simulink model "UpperLimb_Planar"  (R2024b)
settings: Solver=ode45  StartTime=0.0  StopTime=T_sim  FixedStep=1e-3  MaxStep=1e-2  RelTol=1e-3
values from neighbouring files (symbols this model uses):
  activ_dyn = 1    [UpperLimbExo_Parameters.m]
  alpha0 = 180/pi*[M_CORB.alpha0; M_TMAJ.alpha0; M_DELT.alpha0; M_TRIPB.CMED.alpha0; M_TRIPB.CLAT.alpha0;  M_TRIPB.CLONG.alpha0; M_BICB.alpha0; M_BRACH.alpha0]*pi/180    [UpperLimbExo_Parameters.m]
  b12 = dampingOn*0.2    (= 0.2)    [UpperLimbExo_Parameters.m]
  b23 = dampingOn*0.2    (= 0.2)    [UpperLimbExo_Parameters.m]
  FM0 = (1-zraneni).*FM0    [UpperLimbExo_Parameters.m]
  g = 9.81    [UpperLimbExo_Parameters.m]
  I2S2 = 0.0208    [UpperLimbExo_Parameters.m]
  I3S3 = 0.006    [UpperLimbExo_Parameters.m]
  Kd = 2*sqrt(Kp)    [UpperLimbExo_Parameters.m]
  Kp = diag([400, 800])    [UpperLimbExo_Parameters.m]
  Ku = 10    [UpperLimbExo_Parameters.m]
  L2 = 0.29    [UpperLimbExo_Parameters.m]
  LM0 = RATIO.*[M_CORB.LM0; M_TMAJ.LM0; M_DELT.LM0; M_TRIPB.CMED.LM0; M_TRIPB.CLAT.LM0; M_TRIPB.CLONG.LM0; M_BICB.LM0; M_BRACH.LM0]    [UpperLimbExo_Parameters.m]
  LS2 = L2/2    (= 0.145)    [UpperLimbExo_Parameters.m]
  LS3 = LS2    (= 0.145)    [UpperLimbExo_Parameters.m]
  LTs = RATIO.*[M_CORB.LTs; M_TMAJ.LTs; M_DELT.LTs; M_TRIPB.CMED.LTs; M_TRIPB.CLAT.LTs;  M_TRIPB.CLONG.LTs; M_BICB.LTs; M_BRACH.LTs]    [UpperLimbExo_Parameters.m]
  m2 = 2.0519    [UpperLimbExo_Parameters.m]
  m3 = 0.5464 + 0.5464    (= 1.0928)    [UpperLimbExo_Parameters.m]
  T_sampleData = 1e-0    (= 1)    [UpperLimb_Main.m]
  tauA = 15/1000    (= 0.015)    [UpperLimbExo_Parameters.m]
  tauD = 50/1000    (= 0.05)    [UpperLimbExo_Parameters.m]
libraries: simulink_extras x1
settings Model: Creator=jakub  LastModifiedBy=jakub
settings DebuggingCC: ReadBeforeWriteMsg=DisableAll  WriteAfterWriteMsg=DisableAll  WriteAfterReadMsg=DisableAll  MultiTaskDSMMsg=none
settings ModelReferenceCC: UpdateModelReferenceTargets=IfOutOfDate
settings SFSimCC: SFSimEcho=off

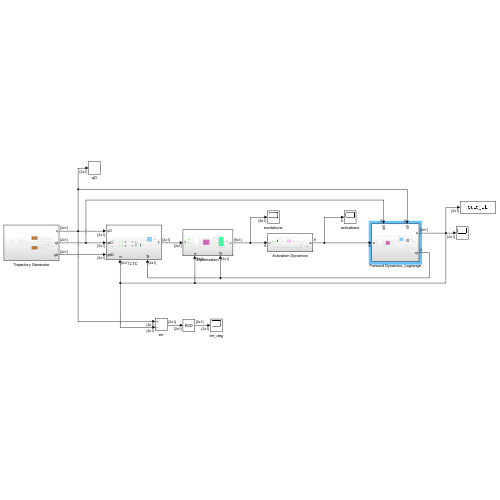
[thumbnail: Simulink's stored preview of the top-level diagram]
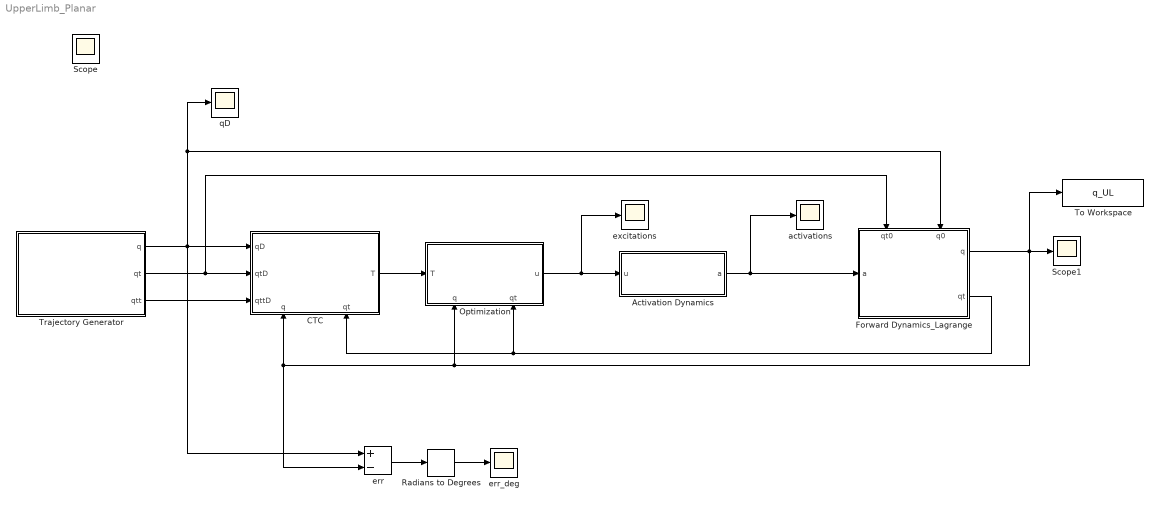
== system UpperLimb_Planar ==
  Activation Dynamics : Subsystem
  CTC : Subsystem
      settings: PortSchema="{\"entries\":[{\"content\":{\"sides\":[{\"content\":{\"connectorIds\":[\"In1\",\"In2\",\"In3\"]},\"type\":\"ConnectorPlacement.EquallySpacedRectSide\",\"uuid\":\"9771eba7-c940-48d8-8da9-6d911b5851fc\"},{\"content\":{\"connectorIds\":[\"Out1\"],\"side\":\"RIGHT\"},\"type\":\"ConnectorPlacement.EquallySpacedRectSide\",\"uuid\":\"6a59c5b5-9e25-411a-90e6-5bf21983ac5c\"},{\"content\":{\"side\":\"TOP\"},\"type\":\"ConnectorPlacement.EquallySpacedRectSide\",\"uuid\":\"c119b971-ed02-4623-8220-b75198a2fdb0\"},{\"content\":{\"connectorIds\":[\"In4\",\"In5\"],\"side\":\"BOTTOM\"},\"type\":\"ConnectorPlacement.EquallySpacedRectSide\",\"uuid\":\"c8357dcf-0796-45f4-b88a-26b4637402a4\"}]},\"type\":\"ConnectorPlacement.EquallySpacedConnector\",\"uuid\":\"a7be367e-b174-4db7-82d5-13ec9cf2ed48\"}],\"packageUris\":[\"http://schema.mathworks.com/mf0/Connector/R2020b\"],\"version\":\"1.0\"}"
  Forward Dynamics_Lagrange : Subsystem
      settings: PortSchema="{\"entries\":[{\"content\":{\"sides\":[{\"content\":{\"connectorIds\":[\"In1\"]},\"type\":\"ConnectorPlacement.EquallySpacedRectSide\",\"uuid\":\"4e4f4804-ca43-420b-a896-94143398389c\"},{\"content\":{\"connectorIds\":[\"Out1\",\"Out2\"],\"side\":\"RIGHT\"},\"type\":\"ConnectorPlacement.EquallySpacedRectSide\",\"uuid\":\"5fd0c042-4ed2-4608-8a89-d3cfef128ff0\"},{\"content\":{\"connectorIds\":[\"In2\",\"In3\"],\"side\":\"TOP\"},\"type\":\"ConnectorPlacement.EquallySpacedRectSide\",\"uuid\":\"9152b886-03a6-40db-8757-3e13ff02ab8e\"},{\"content\":{\"side\":\"BOTTOM\"},\"type\":\"ConnectorPlacement.EquallySpacedRectSide\",\"uuid\":\"2e772fd2-4f40-44b3-932b-1325c76caf16\"}]},\"type\":\"ConnectorPlacement.EquallySpacedConnector\",\"uuid\":\"c9c97ee9-fbd0-4586-b58c-f13fd24f0fc7\"}],\"packageUris\":[\"http://schema.mathworks.com/mf0/Connector/R2020b\"],\"version\":\"1.0\"}"
  Optimization : Subsystem
      settings: PortSchema="{\"entries\":[{\"content\":{\"sides\":[{\"content\":{\"connectorIds\":[\"In1\"]},\"type\":\"ConnectorPlacement.EquallySpacedRectSide\",\"uuid\":\"b44a492b-355a-41d1-979d-356380411af8\"},{\"content\":{\"connectorIds\":[\"Out1\"],\"side\":\"RIGHT\"},\"type\":\"ConnectorPlacement.EquallySpacedRectSide\",\"uuid\":\"d99b47b0-e23d-4c30-9cd9-10c88a2db076\"},{\"content\":{\"side\":\"TOP\"},\"type\":\"ConnectorPlacement.EquallySpacedRectSide\",\"uuid\":\"52778e40-0bc9-47fa-bb22-aef647873746\"},{\"content\":{\"connectorIds\":[\"In2\",\"In3\"],\"side\":\"BOTTOM\"},\"type\":\"ConnectorPlacement.EquallySpacedRectSide\",\"uuid\":\"29328456-4ee0-4f69-ade8-350b50f8103c\"}]},\"type\":\"ConnectorPlacement.EquallySpacedConnector\",\"uuid\":\"e5ef0993-fdc7-4811-bff5-ccf29bcab6f8\"}],\"packageUris\":[\"http://schema.mathworks.com/mf0/Connector/R2020b\"],\"version\":\"1.0\"}"
  Radians to Degrees : simulink_extras/Transformations/Radians to Degrees
  Scope1 : Scope
  To Workspace : ToWorkspace  VariableName=q_UL  SaveFormat=Timeseries  SampleTime=T_sampleData
  Trajectory Generator : Subsystem
  activations : Scope
  err : Sum  Inputs=+-
  err_deg : Scope
  excitations : Scope
  qD : Scope
  Scope : Scope
  wires:
  Optimization/1(u) -> Activation Dynamics/1(u), excitations/1
  CTC/1(T) -> Optimization/1(T)
  Trajectory Generator/1(q) -> CTC/1(qD), err/1, qD/1, Forward Dynamics_Lagrange/3(q0)
  Trajectory Generator/2(qt) -> CTC/2(qtD), Forward Dynamics_Lagrange/2(qt0)
  Trajectory Generator/3(qtt) -> CTC/3(qttD)
  err/1 -> Radians to Degrees/1
  Radians to Degrees/1 -> err_deg/1
  Forward Dynamics_Lagrange/1(q) -> Optimization/2(q), CTC/4(q), err/2, To Workspace/1, Scope1/1
  Forward Dynamics_Lagrange/2(qt) -> Optimization/3(qt), CTC/5(qt)
  Activation Dynamics/1(a) -> activations/1, Forward Dynamics_Lagrange/1(a)

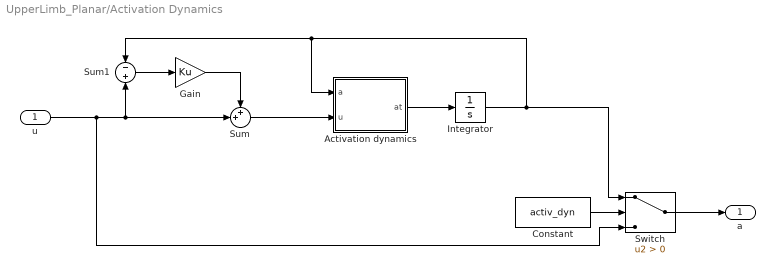
== system UpperLimb_Planar/Activation Dynamics ==
  u : Inport  OutMin=0  OutMax=1  OutDataTypeStr=double  PortDimensions=8  SampleTime=0
  Activation dynamics : MATLAB Function  TreatAsAtomicUnit=on
  Constant : Constant  Value=activ_dyn
  Gain : Gain  Gain=Ku
  Integrator : Integrator  UpperSaturationLimit=1  LowerSaturationLimit=0
  Sum : Sum  Inputs=++|
  Sum1 : Sum  Inputs=-|+
  Switch : Switch  Criteria=u2 > Threshold  ZeroCross=off  SaturateOnIntegerOverflow=off  InputSameDT=off
  a : Outport  OutMin=0  OutMax=1  OutDataTypeStr=double  PortDimensions=8  SampleTime=0
  wires:
  Sum/1 -> Activation dynamics/2(u)
  Integrator/1 -> Switch/1, Sum1/1, Activation dynamics/1(a)
  u/1 -> Sum/2, Sum1/2, Switch/3
  Constant/1 -> Switch/2
  Activation dynamics/1(at) -> Integrator/1
  Switch/1 -> a/1
  Sum1/1 -> Gain/1
  Gain/1 -> Sum/1

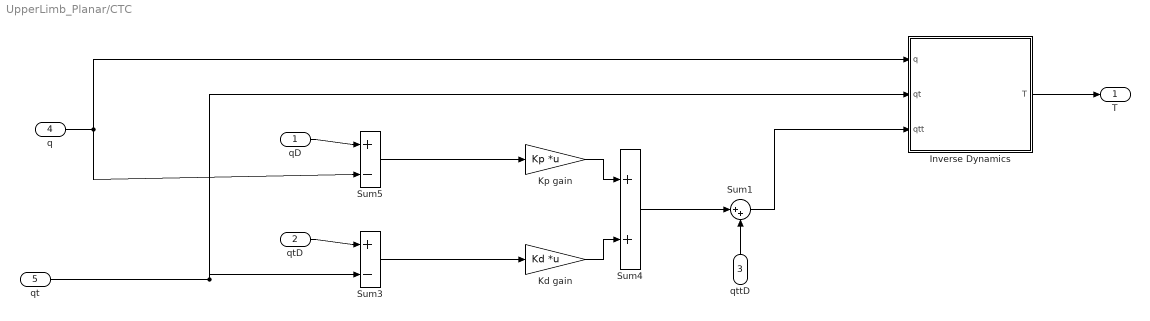
== system UpperLimb_Planar/CTC ==
  qD : Inport  OutDataTypeStr=double  Unit=rad  PortDimensions=[2 1]  SampleTime=0
  qtD : Inport  Port=2  OutDataTypeStr=double  Unit=rad/s  PortDimensions=[2 1]  SampleTime=0
  qttD : Inport  Port=3  OutDataTypeStr=double  Unit=rad/s^2  PortDimensions=[2 1]  SampleTime=0
  q : Inport  Port=4  OutDataTypeStr=double  Unit=rad  PortDimensions=[2 1]  SampleTime=0
  qt : Inport  Port=5  OutDataTypeStr=double  Unit=rad/s  PortDimensions=[2 1]  SampleTime=0
  Inverse Dynamics : MATLAB Function  TreatAsAtomicUnit=on
  Kd gain : Gain  Gain=Kd  Multiplication=Matrix(K*u)  OutDataTypeStr=double
  Kp gain : Gain  Gain=Kp  Multiplication=Matrix(K*u)  OutDataTypeStr=double
  Sum1 : Sum  Inputs=|++  OutDataTypeStr=double
  Sum3 : Sum  Inputs=+|-  OutDataTypeStr=double
  Sum4 : Sum  OutDataTypeStr=double
  Sum5 : Sum  Inputs=+|-  OutDataTypeStr=double
  T : Outport  OutDataTypeStr=double  Unit=N*m  PortDimensions=[2 1]  SampleTime=0
  wires:
  q/1 -> Inverse Dynamics/1(q), Sum5/2
  Inverse Dynamics/1(T) -> T/1
  Sum1/1 -> Inverse Dynamics/3(qtt)
  qttD/1 -> Sum1/2
  Sum5/1 -> Kp gain/1
  Sum4/1 -> Sum1/1
  Kp gain/1 -> Sum4/1
  Sum3/1 -> Kd gain/1
  Kd gain/1 -> Sum4/2
  qD/1 -> Sum5/1
  qtD/1 -> Sum3/1
  qt/1 -> Inverse Dynamics/2(qt), Sum3/2

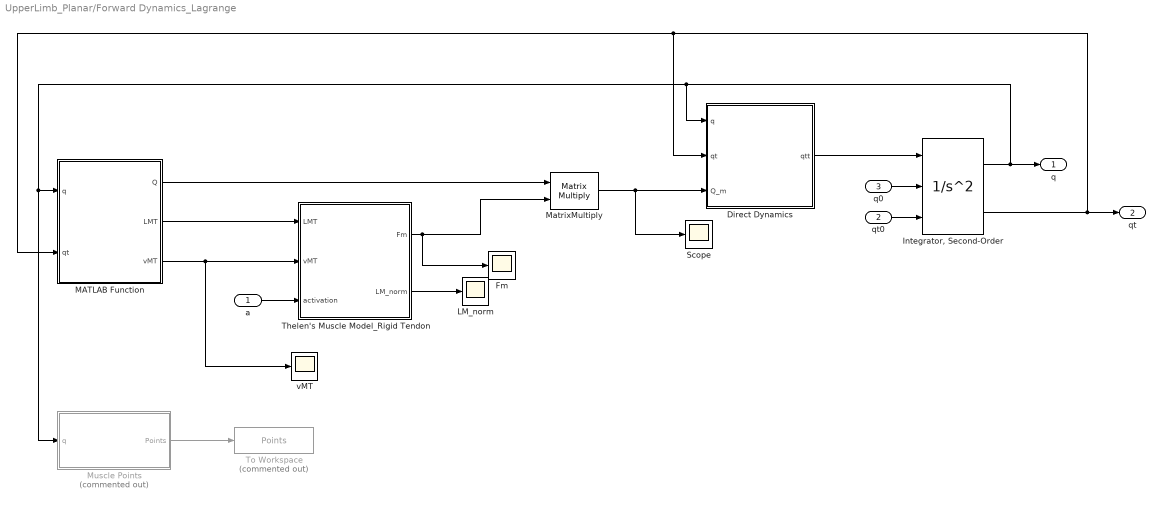
== system UpperLimb_Planar/Forward Dynamics_Lagrange ==
  a : Inport  OutMin=0  OutMax=1  OutDataTypeStr=double  PortDimensions=8  SampleTime=0
  qt0 : Inport  Port=2  OutDataTypeStr=double  Unit=rad/s  PortDimensions=2  SampleTime=0
  q0 : Inport  Port=3  OutDataTypeStr=double  Unit=rad  PortDimensions=2  SampleTime=0
  Direct Dynamics : MATLAB Function  TreatAsAtomicUnit=on
  Fm : Scope
  "Integrator, Second-Order" : SecondOrderIntegrator  ICSourceX=external  ICSourceDXDT=external
  LM_norm : Scope
  MATLAB Function : MATLAB Function  TreatAsAtomicUnit=on
  MatrixMultiply : Product  Multiplication=Matrix(*)  OutDataTypeStr=double
  Muscle Points : MATLAB Function  Commented=on  TreatAsAtomicUnit=on
  Scope : Scope
  Thelen's Muscle Model_Rigid Tendon : MATLAB Function  TreatAsAtomicUnit=on
  To Workspace : ToWorkspace  Commented=on  VariableName=Points  SaveFormat=Timeseries  SampleTime=T_sampleData
  vMT : Scope
  q : Outport  OutDataTypeStr=double  Unit=rad  PortDimensions=[2 1]  SampleTime=0
  qt : Outport  Port=2  OutDataTypeStr=double  Unit=rad/s  PortDimensions=2  SampleTime=0
  wires:
  Direct Dynamics/1(qtt) -> "Integrator, Second-Order"/1
  "Integrator, Second-Order"/2 -> MATLAB Function/2(qt), Direct Dynamics/2(qt), qt/1
  "Integrator, Second-Order"/1 -> q/1, Muscle Points/1(q), MATLAB Function/1(q), Direct Dynamics/1(q)
  qt0/1 -> "Integrator, Second-Order"/3
  q0/1 -> "Integrator, Second-Order"/2
  MATLAB Function/3(vMT) -> Thelen's Muscle Model_Rigid Tendon/2(vMT), vMT/1
  MatrixMultiply/1 -> Scope/1, Direct Dynamics/3(Q_m)
  a/1 -> Thelen's Muscle Model_Rigid Tendon/3(activation)
  Thelen's Muscle Model_Rigid Tendon/2(LM_norm) -> LM_norm/1
  Thelen's Muscle Model_Rigid Tendon/1(Fm) -> MatrixMultiply/2, Fm/1
  MATLAB Function/2(LMT) -> Thelen's Muscle Model_Rigid Tendon/1(LMT)
  MATLAB Function/1(Q) -> MatrixMultiply/1
  Muscle Points/1(Points) -> To Workspace/1

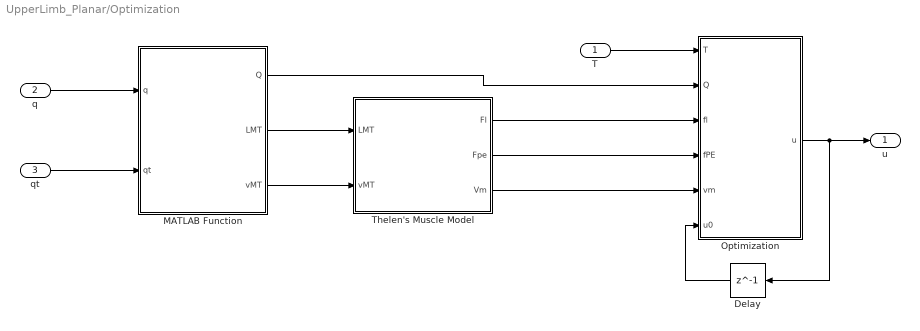
== system UpperLimb_Planar/Optimization ==
  T : Inport  OutDataTypeStr=double  Unit=N*m  PortDimensions=[2 1]  SampleTime=0
  q : Inport  Port=2  OutDataTypeStr=double  Unit=rad  PortDimensions=[2 1]  SampleTime=0
  qt : Inport  Port=3  OutDataTypeStr=double  Unit=rad/sec  PortDimensions=[2 1]  SampleTime=0
  Delay : Delay  DelayLength=1  InitialCondition=0*ones(8,1)
  MATLAB Function : MATLAB Function  TreatAsAtomicUnit=on
  Optimization : MATLAB Function  TreatAsAtomicUnit=on
  Thelen's Muscle Model : MATLAB Function  TreatAsAtomicUnit=on
  u : Outport  OutDataTypeStr=double  PortDimensions=[8 1]  SampleTime=0
  wires:
  Thelen's Muscle Model/3(Vm) -> Optimization/5(vm)
  Thelen's Muscle Model/2(Fpe) -> Optimization/4(fPE)
  MATLAB Function/2(LMT) -> Thelen's Muscle Model/1(LMT)
  MATLAB Function/3(vMT) -> Thelen's Muscle Model/2(vMT)
  qt/1 -> MATLAB Function/2(qt)
  q/1 -> MATLAB Function/1(q)
  Thelen's Muscle Model/1(Fl) -> Optimization/3(fl)
  T/1 -> Optimization/1(T)
  Optimization/1(u) -> Delay/1, u/1
  Delay/1 -> Optimization/6(u0)
  MATLAB Function/1(Q) -> Optimization/2(Q)

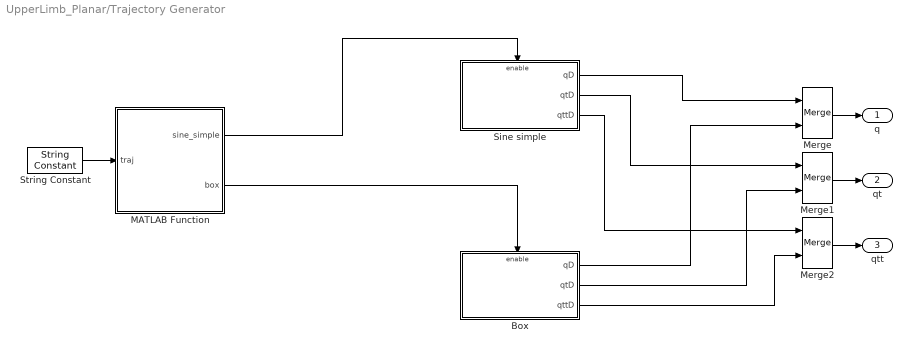
== system UpperLimb_Planar/Trajectory Generator ==
  Box : Subsystem
  MATLAB Function : MATLAB Function  TreatAsAtomicUnit=on
  Merge : Merge
  Merge1 : Merge
  Merge2 : Merge
  Sine simple : Subsystem  TreatAsAtomicUnit=on
  String Constant : StringConstant  String=traj
  q : Outport  OutDataTypeStr=double  Unit=rad  PortDimensions=[2 1]  SampleTime=0
  qt : Outport  Port=2  OutDataTypeStr=double  Unit=rad/sec  PortDimensions=[2 1]  SampleTime=0
  qtt : Outport  Port=3  OutDataTypeStr=double  Unit=rad/s^2  PortDimensions=[2 1]  SampleTime=0
  wires:
  MATLAB Function/2(box) -> Box/Enable
  MATLAB Function/1(sine_simple) -> Sine simple/Enable
  String Constant/1 -> MATLAB Function/1(traj)
  Merge/1 -> q/1
  Sine simple/1(qD) -> Merge/1
  Box/1(qD) -> Merge/2
  Merge1/1 -> qt/1
  Merge2/1 -> qtt/1
  Sine simple/2(qtD) -> Merge1/1
  Box/2(qtD) -> Merge1/2
  Sine simple/3(qttD) -> Merge2/1
  Box/3(qttD) -> Merge2/2

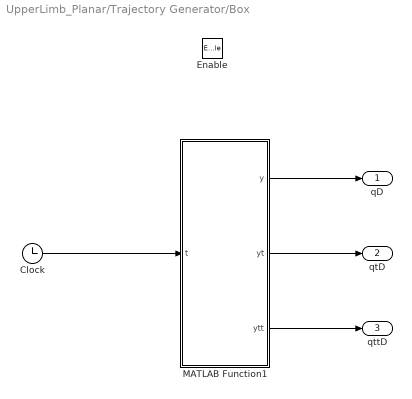
== system UpperLimb_Planar/Trajectory Generator/Box ==
  Enable : EnablePort
  Clock : Clock
  MATLAB Function1 : MATLAB Function  TreatAsAtomicUnit=on
  qD : Outport  OutDataTypeStr=double  Unit=rad  PortDimensions=[2 1]
  qtD : Outport  Port=2  OutDataTypeStr=double  Unit=rad/s  PortDimensions=[2 1]
  qttD : Outport  Port=3  OutDataTypeStr=double  Unit=rad/s^2  PortDimensions=[2 1]
  wires:
  Clock/1 -> MATLAB Function1/1(t)
  MATLAB Function1/1(y) -> qD/1
  MATLAB Function1/2(yt) -> qtD/1
  MATLAB Function1/3(ytt) -> qttD/1

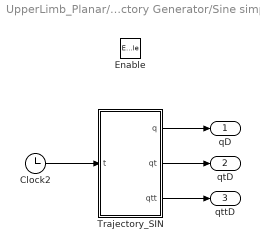
== system UpperLimb_Planar/Trajectory Generator/Sine simple ==
  Enable : EnablePort
  Clock2 : Clock
  Trajectory_SIN : MATLAB Function  TreatAsAtomicUnit=on
  qD : Outport
  qtD : Outport  Port=2
  qttD : Outport  Port=3
  wires:
  Clock2/1 -> Trajectory_SIN/1(t)
  Trajectory_SIN/1(q) -> qD/1
  Trajectory_SIN/2(qt) -> qtD/1
  Trajectory_SIN/3(qtt) -> qttD/1

== matlab function UpperLimb_Planar/Trajectory Generator/Sine simple/Trajectory_SIN ==
  data: t input; q output; qt output; qtt output
function [q, qt, qtt] = fcn(t)

% Trajectory 1
    f1 = 0.5;
    f2 = 0.5;

% % Trajectory 3 - BICB, BRACH injury 90%
%     f1 = 1.3;
%     f2 = 1.3;  

% % REV #3 - response 1Hz
%     f1 = 1;
%     f2 = 1;
% % REV #3 - response 2Hz
%     f1 = 2;
%     f2 = 2;


om1 = 2*pi*f1;
om2 = 2*pi*f2;
psi = -pi/2;


A01 = -pi/4;
A02 = pi/4;
A1 = 0.5*pi/4;
A2 = 0.7*2/4*pi;


fi12 = A01 + A1*sin(om1*t + psi);
fi12t = om1*A1*cos(om1*t + psi);
fi12tt = -om1^2*A1*sin(om1*t + psi);


fi13 = A02 + A2*sin(om2*t + psi);
fi13t = om2*A2*cos(om2*t + psi);
fi13tt = -om2^2*A2*sin(om2*t + psi);

q = [fi12;fi13];
qt = [fi12t;fi13t];
qtt = [fi12tt; fi13tt];

== matlab function UpperLimb_Planar/Forward Dynamics_Lagrange/Thelen's Muscle Model_Rigid Tendon ==
  data: LMT input double size=[8 1]; vMT input double size=[8 1]; Fm output double size=[8 1]; activation input double size=[8 1]; LM0 parameter double size=[8 1]; LTs parameter double size=[8 1]; FM0 parameter double size=[8 1]; alpha0 parameter; LM_norm output
function [Fm, LM_norm]  = Thelen2003(LMT, vMT, activation, LM0, LTs, FM0, alpha0)

    % Muscle constants
        epsM0 = 0.6;            % passive muscle strain due to maximum isometric force
        kPE = 4;                % an exponential shape factor for the passive force-length relationship
        gamma = 0.5;            % a shape factor for the Gaussian active force-length relationship
        Af = 0.3;               % a shape factor for the force-velocity relationship
        fMlen = 1.4;            % maximum normalized muscle force achievable when the fiber is lengthening
        VMmax = 10;


    Fm = zeros(numel(activation),1);
    LM_norm = zeros(numel(activation),1);
    
    for k = 1:numel(LM0)
        Lmt = LMT(k);
        Lt = LTs(k);
        Lm0 = LM0(k);
        Fm0 = FM0(k);
        vmt = vMT(k);
        a = activation(k);
        alpha = alpha0(k);

    %% Muscle length and velocity
        Lm = (Lmt - Lt)/cos(alpha);
        Vm = vmt*cos(alpha);

        lm = Lm/Lm0;

    %% Force of the (contractile element) - ACTIVE FORCE
        fl = exp(-(lm-1)^2/gamma);
        if fl < 0.1
            fl = 0.1;
        end

    %% Force of the muscle parallel element - PASSIVE FORCE
        fpe = (exp(kPE*(lm - 1)/epsM0) - 1) / (exp(kPE) - 1);
        if fpe < 0
            fpe = 0;
        end

    %% Force of the contractile element - Force-velocity relation
        vmmax = VMmax*Lm0;

        if Vm <= 0
            fvm = Af*(4*Vm + vmmax*(3*a + 1)) / (-4*Vm + vmmax*Af*(3*a + 1));
        else
            fvm = (Af*vmmax*(3*a*fMlen - 3*a + fMlen - 1) + 8*Vm*fMlen*(Af + 1)) / (Af*vmmax*(3*a*fMlen - 3*a + fMlen - 1) + 8*Vm*(Af + 1));
        end


    %% Muscle Force
        Fm(k) = Fm0*(a*fl*fvm + fpe)*cos(alpha);

        LM_norm(k) = lm;
    end
        


end

== matlab function UpperLimb_Planar/Optimization/Thelen's Muscle Model ==
  data: LMT input double size=[8 1]; vMT input double size=[8 1]; Fl output double size=[8 1]; LM0 parameter double size=[8 1]; LTs parameter double size=[8 1]; Fpe output double size=[8 1]; Vm output double size=[8 1]; alpha0 parameter
function [Fl, Fpe, Vm]  = Thelen2003(LMT, vMT, LM0, LTs, alpha0)

    % Muscle constants
        epsM0 = 0.6;            % passive muscle strain due to maximum isometric force
        kPE = 4;                % an exponential shape factor for the passive force-length relationship
        gamma = 0.5;            % a shape factor for the Gaussian active force-length relationship

    Fl = zeros(numel(LM0),1);
    Fpe = zeros(numel(LM0),1);
    Vm = zeros(numel(LM0),1);
    
    for k = 1:numel(LM0)
        Lmt = LMT(k);
        Lt = LTs(k);
        Lm0 = LM0(k);
        vmt = vMT(k);
        alpha = alpha0(k);


    %% Muscle length and velocity
        Lm = (Lmt - Lt)/cos(alpha);
        vm = vmt*cos(alpha);

        lm = Lm/Lm0;

    %% Force of the (contractile element) - ACTIVE FORCE
        fl = exp(-(lm-1)^2/gamma);
    
    %% Force of the muscle parallel element - PASSIVE FORCE
        fpe = (exp(kPE*(lm - 1)/epsM0) - 1) / (exp(kPE) - 1);
        if fpe < 0
            fpe = 0;
        end

    %% OUTPUT
        Fpe(k) = fpe;
        Fl(k) = fl;
        Vm(k) = vm;
    end
end

== matlab function UpperLimb_Planar/Optimization/Optimization ==
  data: u output double size=[8 1]; T input double size=[2 1]; Q input double size=[2 8]; fl input double size=[8 1]; fPE input double size=[8 1]; vm input double size=[8 1]; LM0 parameter double size=[8 1]; u0 input double size=[8 1]; alpha0 parameter; FM0 parameter
function u  = fcn(T, Q, fl, fPE, vm, LM0,u0, alpha0, FM0)
u = u0;

% coder.extrinsic('Optimization_ThelenMuscle');
% u = Optimization_ThelenMuscle(Q, T, fl, fPE, vm, LM0, u0, alpha0, FM0);

u = Optimization_ThelenMuscle_codegen(Q, T, fl, fPE, vm, LM0, u0, alpha0, FM0);



end

== matlab function UpperLimb_Planar/Optimization/MATLAB Function ==
  data: Q output; q input; LMT output; qt input; vMT output
function [Q, LMT, vMT] = Muscle_Geometry_ALL(q, qt)

[Q, LMT, vMT] = Muscle_Geometry_ALL(q, qt);

== matlab function UpperLimb_Planar/Activation Dynamics/Activation dynamics ==
  data: a input double size=8 [0..1]; u input double size=8 [0..1]; at output double size=8; tauA parameter double size=1; tauD parameter double size=1
function at = fcn(a,u, tauA, tauD)

at = zeros(numel(u),1);

for k = 1:numel(u)
    if u(k) >= a(k)
        at(k) = (u(k)-a(k))*(u(k)/tauA + (1-u(k))/tauD);
    else
        at(k) = (u(k)-a(k))/tauD;
    end
end

== matlab function UpperLimb_Planar/Trajectory Generator/Box/MATLAB Function1 ==
  data: t input double size=1; y output double size=[2 1]; yt output double size=[2 1]; ytt output double size=[2 1]
function [y,yt,ytt] = fcn(t)

stred12 = (-0.1*pi/2 - 0.9*pi/2)/2;
stred13 = (0.1*pi/2 + 0.7*pi/2)/2;

% Trajectory 2
f = 1;

om = 2*pi*f;
psi = pi/2;

A2 = 0.4*pi/2;
A3 = 0.25*pi/2;

fi12 = stred12 + A2*sin(om*t+psi);
fi12t = A2*om*cos(om*t+psi);
fi12tt = -A2*om^2*sin(om*t+psi);

fi13 = stred13 - A3*sin(om*t+psi);
fi13t = - A3*om*cos(om*t+psi);
fi13tt = + A3*om^2*sin(om*t+psi);



y = [fi12;fi13];
yt = [fi12t; fi13t];
ytt = [fi12tt; fi13tt];

== matlab function UpperLimb_Planar/Forward Dynamics_Lagrange/MATLAB Function ==
  data: Q output; q input; LMT output; qt input; vMT output
function [Q, LMT, vMT] = Muscle_Geometry_ALL(q, qt)

[Q, LMT, vMT] = Muscle_Geometry_ALL(q, qt);

== matlab function UpperLimb_Planar/Forward Dynamics_Lagrange/Muscle Points ==
  data: q input; Points output double
function Points = Muscle_Points_ALL(q)

Points = Muscle_Points_ALL(q);

== matlab function UpperLimb_Planar/Forward Dynamics_Lagrange/Direct Dynamics ==
  data: q input double size=[2 1]; qtt output double size=[2 1]; qt input double size=[2 1]; Q_m input double size=[2 1]; m2 parameter double size=1; m3 parameter double size=1; L2 parameter double size=1; LS2 parameter double size=1; LS3 parameter double size=1; g parameter double size=1; I2S2 parameter double size=1; I3S3 parameter double size=1; b12 parameter double size=1; b23 parameter double size=1
function qtt = fcn(q, qt, Q_m, m2, m3, L2, LS2, LS3, g, I2S2, I3S3, b12, b23)
    G2 = m2*g; G3 = m3*g;

% position, velocity
    fi12 = q(1); fi13 = q(2);
    fi12t = qt(1); fi13t = qt(2);



% Mass Matrix
M = [m2*LS2^2 + I2S2 + m3*L2^2, m3*L2*LS3*cos(fi12 - fi13);
     m3*L2*LS3*cos(fi12 - fi13), m3*LS3^2 + I3S3];

% Corriolis and other acc
H = [fi13t^2*m3*L2*LS3*sin(fi12-fi13);
     -fi12t^2*m3*L2*LS3*sin(fi12-fi13)];

% Gravity forces
Q_g = [-G2*LS2*cos(fi12) - G3*L2*cos(fi12); - G3*LS3*cos(fi13)];

% Damping
Q_b = [-b12*fi12t + b23*(fi13t-fi12t);
       -b23*(fi13t-fi12t)];

Q = Q_g + Q_m + Q_b;

qtt = M\(Q - H);

== matlab function UpperLimb_Planar/Trajectory Generator/MATLAB Function ==
  data: sine_simple output double size=1; box output double size=1; traj input string
function [sine_simple, box] = fcn(traj)

sine_simple = 0;
box = 0;

switch traj
    case "sine_simple"
        sine_simple = 1;

    case "box"
        box = 1;
end

== matlab function UpperLimb_Planar/CTC/Inverse Dynamics ==
  data: q input double size=[2 1]; T output double size=[2 1]; qt input double size=[2 1]; qtt input double size=[2 1]; m2 parameter double size=1; m3 parameter double size=1; L2 parameter double size=1; LS2 parameter double size=1; LS3 parameter double size=1; g parameter double size=1; I2S2 parameter double size=1; I3S3 parameter double size=1; b12 parameter double size=1; b23 parameter double size=1
function T = fcn(q, qt, qtt, m2, m3, L2, LS2, LS3, g, I2S2, I3S3, b12, b23)
    G2 = m2*g; G3 = m3*g;

% position, velocity
    fi12 = q(1); fi13 = q(2);
    fi12t = qt(1); fi13t = qt(2);



% Mass Matrix
M = [m2*LS2^2 + I2S2 + m3*L2^2, m3*L2*LS3*cos(fi12 - fi13);
     m3*L2*LS3*cos(fi12 - fi13), m3*LS3^2 + I3S3];

% Corriolis and other acc
H = [fi13t^2*m3*L2*LS3*sin(fi12-fi13);
     -fi12t^2*m3*L2*LS3*sin(fi12-fi13)];

% Gravity forces
Q_g = [-G2*LS2*cos(fi12) - G3*L2*cos(fi12); - G3*LS3*cos(fi13)];

% Damping
Q_b = [-b12*fi12t + b23*(fi13t-fi12t);
       -b23*(fi13t-fi12t)];

Q = Q_g + Q_b;

T = M*qtt + H - Q;
